simulink model "NewtonsCoolingLaw"  (R2022a)
settings: Solver=VariableStepAuto  StartTime=0.0  StopTime=10.0  RelTol=1e-3
undefined symbols (not defined in the file): k, T0
settings Model: Creator=Adam Ghatta  LastModifiedBy=Adam Ghatta

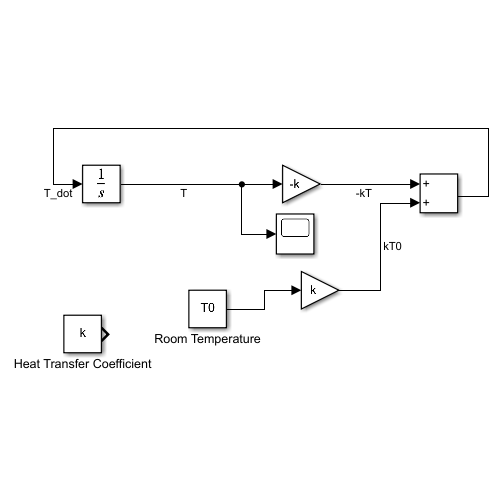
[thumbnail: Simulink's stored preview of the top-level diagram]
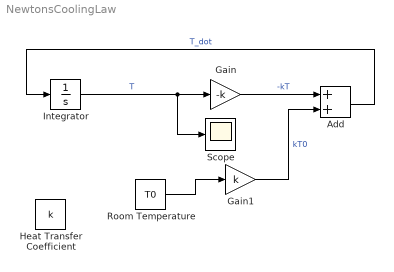
== system NewtonsCoolingLaw ==
  Add : Sum
  Gain : Gain  Gain=-k
  Gain1 : Gain  Gain=k
  Heat Transfer Coefficient : Constant  Value=k
  Integrator : Integrator  InitialCondition=300
  Room Temperature : Constant  Value=T0
  Scope : Scope
  wires:
  Integrator/1 -> Scope/1, Gain/1  "T"
  Add/1 -> Integrator/1  "T_dot"
  Gain/1 -> Add/1  "-kT"
  Room Temperature/1 -> Gain1/1
  Gain1/1 -> Add/2  "kT0"
